simulink model "test_patterns"  (R2014a)
settings: Solver=ode3  StartTime=0.0  StopTime=10.0  RelTol=1e-3
libraries: patterns_library x24
settings Model: Creator=lgwagner  LastModifiedBy=lgwagner

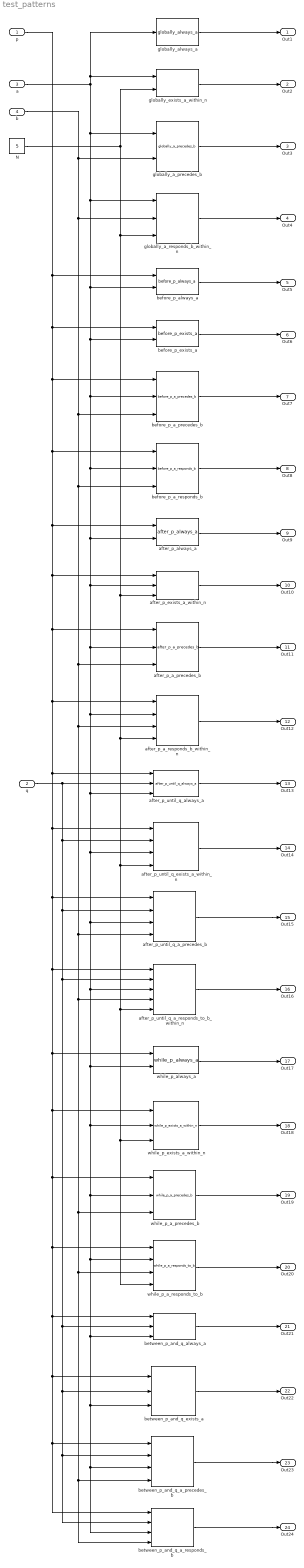
== system test_patterns ==
  p : Inport  OutDataTypeStr=boolean
  q : Inport  Port=2  OutDataTypeStr=boolean
  a : Inport  Port=3  OutDataTypeStr=boolean
  b : Inport  Port=4  OutDataTypeStr=boolean
  N : Constant  Value=5
  after_p_a_precedes_b : patterns_library/after_p_a_precedes_b
  after_p_a_responds_b_within_n : patterns_library/after_p_a_responds_b_within_n
  after_p_always_a : patterns_library/after_p_always_a
  after_p_exists_a_within_n : patterns_library/after_p_exists_a_within_n
  after_p_until_q_a_precedes_b : patterns_library/after_p_until_q_a_precedes_b
  after_p_until_q_a_responds_to_b_within_n : patterns_library/after_p_until_q_a_responds_to_b_within_n
  after_p_until_q_always_a : patterns_library/after_p_until_q_always_a
  after_p_until_q_exists_a_within_n : patterns_library/after_p_until_q_exists_a_within_n
  before_p_a_precedes_b : patterns_library/before_p_a_precedes_b
  before_p_a_responds_b : patterns_library/before_p_a_responds_b
  before_p_always_a : patterns_library/before_p_always_a
  before_p_exists_a : patterns_library/before_p_exists_a
  between_p_and_q_a_precedes_b : patterns_library/between_p_and_q_a_precedes_b
  between_p_and_q_a_responds_b : patterns_library/between_p_and_q_a_responds_b
  between_p_and_q_always_a : patterns_library/between_p_and_q_always_a
  between_p_and_q_exists_a : patterns_library/between_p_and_q_exists_a
  globally_a_precedes_b : patterns_library/globally_a_precedes_b
  globally_a_responds_b_within_n : patterns_library/globally_a_responds_b_within_n
  globally_always_a : patterns_library/globally_always_a
  globally_exists_a_within_n : patterns_library/globally_exists_a_within_n
  while_p_a_precedes_b : patterns_library/while_p_a_precedes_b
  while_p_a_responds_to_b : patterns_library/while_p_a_responds_to_b
  while_p_always_a : patterns_library/while_p_always_a
  while_p_exists_a_within_n : patterns_library/while_p_exists_a_within_n
  Out1 : Outport
  Out2 : Outport  Port=2
  Out3 : Outport  Port=3
  Out4 : Outport  Port=4
  Out5 : Outport  Port=5
  Out6 : Outport  Port=6
  Out7 : Outport  Port=7
  Out8 : Outport  Port=8
  Out9 : Outport  Port=9
  Out10 : Outport  Port=10
  Out11 : Outport  Port=11
  Out12 : Outport  Port=12
  Out13 : Outport  Port=13
  Out14 : Outport  Port=14
  Out15 : Outport  Port=15
  Out16 : Outport  Port=16
  Out17 : Outport  Port=17
  Out18 : Outport  Port=18
  Out19 : Outport  Port=19
  Out20 : Outport  Port=20
  Out21 : Outport  Port=21
  Out22 : Outport  Port=22
  Out23 : Outport  Port=23
  Out24 : Outport  Port=24
  wires:
  b/1 -> globally_a_precedes_b/2, globally_a_responds_b_within_n/2, between_p_and_q_a_precedes_b/4, between_p_and_q_a_responds_b/4, while_p_a_responds_to_b/3, while_p_a_precedes_b/3, after_p_until_q_a_responds_to_b_within_n/4, after_p_until_q_a_precedes_b/4, after_p_a_responds_b_within_n/3, after_p_a_precedes_b/3, before_p_a_responds_b/3, before_p_a_precedes_b/3
  p/1 -> before_p_exists_a/1, before_p_a_precedes_b/1, while_p_exists_a_within_n/1, between_p_and_q_a_responds_b/1, between_p_and_q_a_precedes_b/1, between_p_and_q_exists_a/1, between_p_and_q_always_a/1, while_p_a_responds_to_b/1, while_p_a_precedes_b/1, while_p_always_a/1, after_p_until_q_a_responds_to_b_within_n/1, after_p_until_q_a_precedes_b/1, after_p_until_q_exists_a_within_n/1, after_p_until_q_always_a/1, after_p_a_responds_b_within_n/1, after_p_a_precedes_b/1, after_p_exists_a_within_n/1, after_p_always_a/1, before_p_a_responds_b/1, before_p_always_a/1
  globally_always_a/1 -> Out1/1
  globally_exists_a_within_n/1 -> Out2/1
  globally_a_precedes_b/1 -> Out3/1
  globally_a_responds_b_within_n/1 -> Out4/1
  before_p_always_a/1 -> Out5/1
  before_p_exists_a/1 -> Out6/1
  before_p_a_precedes_b/1 -> Out7/1
  before_p_a_responds_b/1 -> Out8/1
  a/1 -> before_p_exists_a/2, before_p_a_precedes_b/2, after_p_until_q_always_a/3, while_p_always_a/2, while_p_exists_a_within_n/2, while_p_a_responds_to_b/2, between_p_and_q_always_a/3, between_p_and_q_a_responds_b/3, between_p_and_q_a_precedes_b/3, between_p_and_q_exists_a/3, while_p_a_precedes_b/2, after_p_until_q_a_responds_to_b_within_n/3, after_p_until_q_a_precedes_b/3, after_p_until_q_exists_a_within_n/3, after_p_a_responds_b_within_n/2, after_p_a_precedes_b/2, after_p_exists_a_within_n/2, after_p_always_a/2, before_p_a_responds_b/2, before_p_always_a/2, globally_a_responds_b_within_n/1, globally_a_precedes_b/1, globally_exists_a_within_n/1, globally_always_a/1
  N/1 -> after_p_until_q_exists_a_within_n/4, while_p_a_responds_to_b/4, while_p_exists_a_within_n/3, after_p_until_q_a_responds_to_b_within_n/5, after_p_a_responds_b_within_n/4, after_p_exists_a_within_n/3, globally_a_responds_b_within_n/3, globally_exists_a_within_n/2
  after_p_always_a/1 -> Out9/1
  after_p_exists_a_within_n/1 -> Out10/1
  after_p_a_precedes_b/1 -> Out11/1
  after_p_a_responds_b_within_n/1 -> Out12/1
  q/1 -> after_p_until_q_exists_a_within_n/2, after_p_until_q_a_precedes_b/2, after_p_until_q_a_responds_to_b_within_n/2, between_p_and_q_a_responds_b/2, between_p_and_q_a_precedes_b/2, between_p_and_q_exists_a/2, between_p_and_q_always_a/2, after_p_until_q_always_a/2
  after_p_until_q_always_a/1 -> Out13/1
  after_p_until_q_exists_a_within_n/1 -> Out14/1
  after_p_until_q_a_precedes_b/1 -> Out15/1
  after_p_until_q_a_responds_to_b_within_n/1 -> Out16/1
  while_p_always_a/1 -> Out17/1
  while_p_exists_a_within_n/1 -> Out18/1
  while_p_a_precedes_b/1 -> Out19/1
  while_p_a_responds_to_b/1 -> Out20/1
  between_p_and_q_always_a/1 -> Out21/1
  between_p_and_q_exists_a/1 -> Out22/1
  between_p_and_q_a_precedes_b/1 -> Out23/1
  between_p_and_q_a_responds_b/1 -> Out24/1
